simulink model "conttest_discrete"  (Simulink 6.5)
settings: Solver=FixedStepDiscrete  StartTime=0.0  StopTime=max(T)  FixedStep=delta_t  RelTol=1e-3
values from neighbouring files (symbols this model uses):
  delta_t = 1e-4    (= 0.0001)    [makesim.m]    (also in runsim_PID.m)
  Gd = c2d(G,delta_t,'tustin')    [makesim.m]
  Kwredd = c2d(Kwred,delta_t,'tustin')    [makesim.m]
  PSlimits = PSlimits(1:size(K,1))    [makesim.m]
  Wid = c2d(Wi,delta_t,'tustin')    [makesim.m]
  Wod = c2d(Wo,delta_t,'tustin')    [makesim.m]
settings Model: Creator=asharma  LastModifiedBy=asharma  ExtModeTrigMode=oneshot  ExtModeArmWhenConnect=off  ExtModeAutoUpdateStatusClock=off
settings DataIOCC: LimitDataPoints=off
settings OptimizationCC: BooleanDataType=off
settings DebuggingCC: SolverPrmCheckMsg=none  MultiTaskDSMMsg=warning  MultiTaskCondExecSysMsg=none  StrictBusMsg=None
settings HardwareCC: TargetUnknown=on
settings RTWCC: IncludeERTFirstTime=on

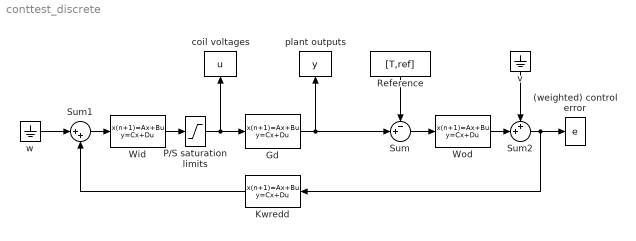
== system conttest_discrete ==
  (weighted) control error : ToWorkspace  VariableName=e  SampleTime=-1  SaveFormat=Array
  Gd : DiscreteStateSpace  A=Gd.A  B=Gd.B  C=Gd.C  D=Gd.D  SampleTime=delta_t
  Kwredd : DiscreteStateSpace  Orientation=left  A=Kwredd.A  B=Kwredd.B  C=Kwredd.C  D=Kwredd.D  SampleTime=delta_t
  P/S saturation limits : Saturate  UpperLimit=PSlimits  LowerLimit=-PSlimits
  Reference : FromWorkspace  Orientation=down  VariableName=[T,ref]  SampleTime=delta_t  Interpolate=off  OutputAfterFinalValue=Setting to zero
  Sum : Sum  Inputs=-+|  SaturateOnIntegerOverflow=on  InputSameDT=on
  Sum1 : Sum  Inputs=|++  SaturateOnIntegerOverflow=on  InputSameDT=on
  Sum2 : Sum  Inputs=++|  SaturateOnIntegerOverflow=on  InputSameDT=on
  Wid : DiscreteStateSpace  A=Wid.A  B=Wid.B  C=Wid.C  D=Wid.D  SampleTime=delta_t
  Wod : DiscreteStateSpace  A=Wod.A  B=Wod.B  C=Wod.C  D=Wod.D  SampleTime=delta_t
  coil voltages : ToWorkspace  VariableName=u  SampleTime=-1  SaveFormat=Array
      settings: Orientation=up
  plant outputs : ToWorkspace  VariableName=y  SampleTime=-1  SaveFormat=Array
      settings: Orientation=up
  v : Ground  Orientation=down
  w : Ground
  wires:
  Wid/1 -> P/S saturation limits/1
  w/1 -> Sum1/1
  Sum1/1 -> Wid/1
  Reference/1 -> Sum/1
  Gd/1 -> plant outputs/1, Sum/2
  P/S saturation limits/1 -> Gd/1, coil voltages/1
  Sum/1 -> Wod/1
  Wod/1 -> Sum2/2
  v/1 -> Sum2/1
  Sum2/1 -> (weighted) control error/1, Kwredd/1
  Kwredd/1 -> Sum1/2
